simulink model "siso_4_channel_teleop_discrete_wave_PosPos_noise"  (R2021a)
settings: Solver=VariableStepAuto  StartTime=0.0  StopTime=30  FixedStep=Ts  RelTol=1e-3
values from neighbouring files (symbols this model uses):
  A_kalman = [1 Ts ; 0 1 ]    [assignment6.m]
  Amplitude = 1    [assignment6.m]
  b = 1    [assignment6.m]    (also in lessonParams.m)
  Be = 10    [assignment6.m]    (also in lessonParams.m)
  Bh = 1.5    [assignment6.m]    (also in lessonParams.m)
  Bm = 10    [assignment6.m]
  Bs = 30    [assignment6.m]
  C_kalman = [1 0]    [assignment6.m]
  delay = 20    [assignment6.m]
  Dh = 2    [assignment6.m]    (also in lessonParams.m)
  Dm = 0    [assignment6.m]
  Ds = 0    [assignment6.m]
  Fc = 0.1    [assignment6.m]    (also in lessonParams.m = 1)
  Flp = 5    [assignment6.m]
  Ih = 0    [assignment6.m]
  Jh = 0    [assignment6.m]    (also in lessonParams.m = 0.05)
  k_h = 2    [assignment6.m]
  Ke = 200    [assignment6.m]    (also in lessonParams.m)
  Kh = 1    [assignment6.m]    (also in lessonParams.m = 0)
  Km = 50    [assignment6.m]
  Ks = 40    [assignment6.m]
  Mm = 0.5    [assignment6.m]
  Ms = 2    [assignment6.m]
  noiseVariance = 0.00001    (= 1e-05)    [assignment6.m]
  R = 1    [assignment6.m]
  Ts = 0.001    [assignment6.m]    (also in lessonParams.m)
  xe = 0.65    [assignment6.m]
undefined symbols (not defined in the file or in its folder): B, D, DiscIntNeverNeededParam, Discrete, Time
libraries: simulink x4, ctrlSharedLib x2
settings Model: Creator=fabio  LastModifiedBy=fabio

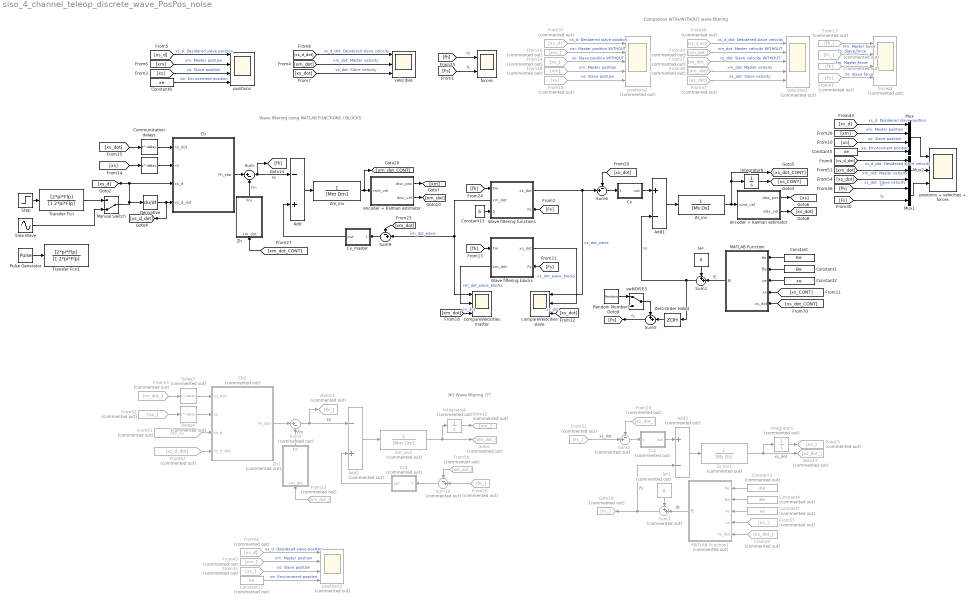
== system siso_4_channel_teleop_discrete_wave_PosPos_noise ==
  note: Wave filtering using MATLAB FUNCTIONS / BLOCKS
  note: Comparison WITH/WITHOUT wave filtering
  note: NO Wave filtering ???
  " " : Delay  DelayLength=delay  SampleTime=Ts
  Add : Sum  Inputs=-+
  Add1 : Sum  Inputs=+-
  Add2 : Sum  Commented=on  Inputs=-+
  Add3 : Sum  Commented=on  Inputs=+-
  Ch : Subsystem
  Ch2 : Subsystem  Commented=on
  Communication delays : Delay  DelayLength=delay  SampleTime=Ts
  Constant : Constant  Value=Ke
  Constant1 : Constant  Value=Be
  Constant11 : Constant  Commented=on  Value=xe
  Constant13 : Constant  Value=b
  Constant2 : Constant  Value=xe
  Constant3 : Constant  Commented=on  Value=Ke
  Constant4 : Constant  Commented=on  Value=Be
  Constant5 : Constant  Value=xe
  Constant6 : Constant  Value=xe
  Constant7 : Constant  Commented=on  Value=xe
  Cv : Subsystem
  Cv1 : Subsystem  Commented=on
  Cv4 : Subsystem  Commented=on
  Cv_master : Subsystem
  Delay3 : Delay  Commented=on  DelayLength=delay  SampleTime=Ts
  Delay4 : Delay  Commented=on  DelayLength=delay  SampleTime=Ts
  Derivative : Derivative
  From17 : From  Commented=on  GotoTag=fh_
  From18 : From  Commented=on  GotoTag=xs
  From{19,29,37,53} (4 alike) : From  Commented=on  GotoTag=xs_dot_
  From22 : From  Commented=on  GotoTag=xm_dot_
  From26 : From  Commented=on  GotoTag=fh_
  From31 : From  Commented=on  GotoTag=Fs_
  From32 : From  Commented=on  GotoTag=Fs_
  From{33..34,52,55} (4 alike) : From  Commented=on  GotoTag=xs_
  From35 : From  Commented=on  GotoTag=xs_d
  From36 : From  Commented=on  GotoTag=xm_
  From38 : From  Commented=on  GotoTag=xm
  From39 : From  Commented=on  GotoTag=xm_dot_
  From40 : From  Commented=on  GotoTag=fh
  From41 : From  Commented=on  GotoTag=Fs
  From42 : From  Commented=on  GotoTag=xs_d
  From45 : From  Commented=on  GotoTag=xm_
  From47 : From  Commented=on  GotoTag=xs_dot
  From48 : From  Commented=on  GotoTag=xs_d_dot
  From49 : From  Commented=on  GotoTag=xm_dot
  From50 : From  Commented=on  GotoTag=xm_dot_
  From61 : From  Commented=on  GotoTag=xs_d
  From62 : From  Commented=on  GotoTag=xs_d_dot
  Goto1 : Goto  Commented=on  GotoTag=xm_dot_
  Goto11 : Goto  Commented=on  GotoTag=fh_
  Goto12 : Goto  Commented=on  GotoTag=xm_
  Goto15 : Goto  Commented=on  GotoTag=xs_
  Goto17 : Goto  Commented=on  GotoTag=xs_dot_
  Goto18 : Goto  Commented=on  GotoTag=Fs_
  Integrator1 : Integrator  Commented=on
  Integrator4 : Integrator  Commented=on
  Integrator6 : Integrator
  MATLAB Function : MATLAB Function  TreatAsAtomicUnit=on
  MATLAB Function1 : MATLAB Function  Commented=on  TreatAsAtomicUnit=on
  Manual Switch : ManualSwitch  CurrentSetting=0
  Mux : Mux
  Mux1 : Mux  Inputs=2
  Mux2 : Mux  Inputs=3
  Pulse Generator : DiscretePulseGenerator  PulseType=Time based  Amplitude=Amplitude  PulseWidth=50  PhaseDelay=1
  Random Number1 : RandomNumber  Variance=noiseVariance  SampleTime=Ts
  Sine Wave : Sin  Amplitude=Amplitude  Frequency=Fc*2*pi  SampleTime=0
  Step : Step  After=Amplitude  SampleTime=0
  Sum : Sum  Inputs=|+-
  Sum1 : Sum  Inputs=++|
  Sum10 : Sum  Commented=on  Inputs=-+|
  Sum2 : Sum  Commented=on  Inputs=|+-
  Sum3 : Sum  Commented=on  Inputs=++|
  Sum4 : Sum  Commented=on  Inputs=-+|
  Sum5 : Sum  Inputs=++|
  Sum6 : Sum  Inputs=-+|
  Sum9 : Sum  Inputs=-+|
  Transfer Fcn : TransferFcn  Numerator=[2*pi*Flp]  Denominator=[1 2*pi*Flp]
  Transfer Fcn1 : TransferFcn  Numerator=[2*pi*Flp]  Denominator=[1 2*pi*Flp]
  Wave filtering blocks : Subsystem
      settings: PortSchema="{\"entries\":[{\"content\":{\"sides\":[{\"content\":{\"connectorIds\":[\"In1\",\"Out2\"]},\"type\":\"ConnectorPlacement.EquallySpacedRectSide\",\"uuid\":\"ee55f81f-a118-497c-9cea-fc8f399218a8\"},{\"content\":{\"connectorIds\":[\"Out1\",\"In2\"],\"side\":\"RIGHT\"},\"type\":\"ConnectorPlacement.EquallySpacedRectSide\",\"uuid\":\"5d1f8501-e1f6-44bf-840d-44d9be1b0103\"},{\"content\":{\"connectorIds\":[],\"side\":\"TOP\"},\"type\":\"ConnectorPlacement.EquallySpacedRectSide\",\"uuid\":\"9e5e7cf5-c9c8-426d-b3a0-7ec1f0160b8f\"}]},\"type\":\"ConnectorPlacement.EquallySpacedConnector\",\"uuid\":\"44941e1b-3958-484a-ae3c-a91d5c4b8d1b\"}],\"packageUris\":[\"http://schema.mathworks.com/mf0/Connector/R2020b\"],\"version\":\"1.0\"}"
  "Wave filtering functions " : Subsystem
      settings: PortSchema="{\"entries\":[{\"content\":{\"sides\":[{\"content\":{\"connectorIds\":[\"In1\",\"Out2\",\"In2\"]},\"type\":\"ConnectorPlacement.EquallySpacedRectSide\",\"uuid\":\"83e83ea2-dad7-4848-b95e-28bc67907647\"},{\"content\":{\"connectorIds\":[\"Out1\",\"In3\"],\"side\":\"RIGHT\"},\"type\":\"ConnectorPlacement.EquallySpacedRectSide\",\"uuid\":\"35e14d6e-ed23-456f-ac9f-64c013712c68\"},{\"content\":{\"connectorIds\":[],\"side\":\"TOP\"},\"type\":\"ConnectorPlacement.EquallySpacedRectSide\",\"uuid\":\"299d1efd-7af2-45ae-8d8e-9fad00b289c8\"}]},\"type\":\"ConnectorPlacement.EquallySpacedConnector\",\"uuid\":\"2f111283-4845-4b8e-bf59-fc37d8c45372\"}],\"packageUris\":[\"http://schema.mathworks.com/mf0/Connector/R2020b\"],\"version\":\"1.0\"}"
  Zero-Order Hold4 : ZeroOrderHold  SampleTime=Ts
  Zh : Subsystem
  Zh1 : Subsystem  Commented=on
  Zm_inv : TransferFcn  Numerator=[0 1]  Denominator=[Mm Dm]
  Zm_inv1 : TransferFcn  Commented=on  Numerator=[0 1]  Denominator=[Mm Dm]
  Zs_inv : TransferFcn  Numerator=[0 1]  Denominator=[Ms Ds]
  Zs_inv1 : TransferFcn  Commented=on  Numerator=[0 1]  Denominator=[Ms Ds]
  "compareVelocities master " : Scope  NumInputPorts=3
  compareVelocities slave : Scope  NumInputPorts=3
  encoder + Kalman estimator : Subsystem
  "encoder + Kalman estimator " : Subsystem
  fe* : Constant  Value=0
  fe*1 : Constant  Commented=on  Value=0
  forces : Scope  NumInputPorts=2
  forces2 : Scope  Commented=on  NumInputPorts=4
  positions : Scope  NumInputPorts=4
  positions + velocities + forces : Scope  NumInputPorts=3
  positions1 : Scope  Commented=on  NumInputPorts=4
  positions2 : Scope  Commented=on  NumInputPorts=5
  swNOISE3 : ManualSwitch
  velocities : Scope  NumInputPorts=3
  velocities1 : Scope  Commented=on  NumInputPorts=5
  wires:
  Zh/1(Fm) -> Sum/2  "Fm"
  Sum/1 -> Add/1, [fh]  "Fh"
  Constant/1 -> MATLAB Function/1(Ke)
  Constant1/1 -> MATLAB Function/2(Be)
  Constant2/1 -> MATLAB Function/3(xe)
  [xs_CONT] -> MATLAB Function/4(xs)
  [xs_dot_CONT] -> MATLAB Function/5(xs_dot)
  MATLAB Function/1(fE) -> Sum1/2  "fE"
  Cv/1(out) -> Add1/1
  Ch/1(Fh_star) -> Sum/1
  [xs_d] -> positions/1  "xs_d: Desidered slave position"
  [xm] -> positions/2  "xm: Master position"
  [xs] -> positions/3  "xs: Slave position"
  [xm_dot] -> velocities/2  "xm_dot: Master velocity"
  [xs_dot] -> velocities/3  "xs_dot: Slave velocity"
  [xs_d_dot] -> velocities/1  "xs_d_dot: Desidered slave velocity"
  Sine Wave/1 -> Manual Switch/2
  Derivative/1 -> [xs_d_dot], Ch/1(xs_d_dot)
  fe*/1 -> Sum1/1
  Step/1 -> Transfer Fcn/1
  Transfer Fcn/1 -> Manual Switch/1
  Manual Switch/1 -> Ch/2(xs_d), [xs_d], Derivative/1
  [xm_dot_CONT] -> Zh/1(xm_dot)
  Constant6/1 -> positions/4  "xe: Environment position"
  [fh] -> forces/1  "fh"
  [Fs] -> forces/2  "fs"
  Pulse Generator/1 -> Transfer Fcn1/1
  [xs_dot] -> Communication delays/1
  Communication delays/1 -> Ch/4(xs_dot)
  [xs] -> " "/1
  " "/1 -> Ch/3(xs)
  [xs_dot] -> Sum6/1
  Sum6/1 -> Cv/1(velErr)
  [xs_dot] -> compareVelocities slave/3  "xs_dot"
  From48/1 -> velocities1/1  "xs_d_dot: Desidered slave velocity"
  From47/1 -> velocities1/5  "xs_dot: Slave velocity"
  From17/1 -> forces2/1  "Fm: Master force"
  From37/1 -> velocities1/3  "xs_dot: Slave velocity WITHOUT"
  From39/1 -> velocities1/2  "xm_dot: Master velocity WITHOUT"
  From40/1 -> forces2/3  "Fm: Master force"
  From18/1 -> positions2/5  "xs: Slave position"
  From35/1 -> positions2/1  "xs_d: Desidered slave position"
  From49/1 -> velocities1/4  "xm_dot: Master velocity"
  From32/1 -> forces2/2  "Fs: Slave force"
  From34/1 -> positions2/3  "xs: Slave position WITHOUT"
  From38/1 -> positions2/4  "xm: Master position"
  From36/1 -> positions2/2  "xm: Master position WITHOUT"
  From41/1 -> forces2/4  "Fs: Slave force"
  Constant11/1 -> positions1/4  "xe: Environment position"
  From33/1 -> positions1/3  "xs: Slave position"
  From45/1 -> positions1/2  "xm: Master position"
  From42/1 -> positions1/1  "xs_d: Desidered slave position"
  Sum1/1 -> Add1/2, Zero-Order Hold4/1  "Fs"
  Sum9/1 -> Cv_master/1(velErr)
  [xm_dot] -> Sum9/1
  [Fs] -> "Wave filtering functions "/3(Fs)
  [fh] -> "Wave filtering functions "/1(Fm)
  Cv_master/1(out) -> Add/2
  Constant13/1 -> "Wave filtering functions "/2(b)
  [fh] -> Wave filtering blocks/1(Fm)
  [Fs] -> Wave filtering blocks/2(Fs)
  Wave filtering blocks/1(xs_dot) -> compareVelocities slave/2  "xs_dot_wave_blocks"
  Wave filtering blocks/2(xm_dot) -> "compareVelocities master "/2  "xm_dot_wave_blocks"
  "Wave filtering functions "/2(xm_dot) -> Sum9/2, "compareVelocities master "/1  "xm_dot_wave"
  "Wave filtering functions "/1(xs_dot) -> Sum6/2, compareVelocities slave/1  "xs_dot_wave"
  From55/1 -> MATLAB Function1/4(xs)
  Integrator1/1 -> Goto15/1
  Cv4/1(out) -> Add2/2
  Ch2/1(Fh_star) -> Sum2/1
  From50/1 -> Sum10/1
  Sum3/1 -> Add3/2, Goto18/1  "Fs"
  From29/1 -> Sum4/1
  Constant7/1 -> MATLAB Function1/3(xe)
  Sum10/1 -> Cv4/1(velErr)
  Sum2/1 -> Add2/1, Goto11/1  "Fh"
  Zm_inv1/1 -> Integrator4/1, Goto1/1
  Cv1/1(out) -> Add3/1
  From19/1 -> MATLAB Function1/5(xs_dot)
  Add3/1 -> Zs_inv1/1
  Add2/1 -> Zm_inv1/1
  Zh1/1(Fm) -> Sum2/2  "Fm"
  Constant3/1 -> MATLAB Function1/1(Ke)
  MATLAB Function1/1(fE) -> Sum3/2  "fE"
  Sum4/1 -> Cv1/1(velErr)
  Constant4/1 -> MATLAB Function1/2(Be)
  Integrator4/1 -> Goto12/1
  From22/1 -> Zh1/1(xm_dot)
  Zs_inv1/1 -> Goto17/1, Integrator1/1  "xs_dot"
  fe*1/1 -> Sum3/1
  Delay3/1 -> Ch2/4(xs_dot)
  From52/1 -> Delay4/1
  From61/1 -> Ch2/2(xs_d)
  From53/1 -> Delay3/1
  Delay4/1 -> Ch2/3(xs)
  From62/1 -> Ch2/1(xs_d_dot)
  From26/1 -> Sum10/2
  From31/1 -> Sum4/2  "xs_dot"
  Add/1 -> Zm_inv/1
  Zm_inv/1 -> [xm_dot_CONT], encoder + Kalman estimator/1(cont_vel)
  encoder + Kalman estimator/1(disc_pos) -> [xm]
  encoder + Kalman estimator/2(disc_vel) -> [xm_dot]
  "encoder + Kalman estimator "/2(disc_vel) -> [xs_dot]
  Integrator6/1 -> [xs_CONT]
  Zs_inv/1 -> Integrator6/1, [xs_dot_CONT], "encoder + Kalman estimator "/1(cont_vel)
  Add1/1 -> Zs_inv/1
  "encoder + Kalman estimator "/1(disc_pos) -> [xs]
  swNOISE3/1 -> Sum5/1
  Random Number1/1 -> swNOISE3/1
  Zero-Order Hold4/1 -> Sum5/2
  Sum5/1 -> [Fs]  "fs"
  [xm_dot] -> "compareVelocities master "/3  "xm_dot"
  Mux1/1 -> positions + velocities + forces/3
  [xs_d_dot] -> Mux2/1  "xs_d_dot: Desidered slave velocity"
  Constant5/1 -> Mux/4  "xe: Environment position"
  Mux/1 -> positions + velocities + forces/1
  Mux2/1 -> positions + velocities + forces/2
  [fh] -> Mux1/1  "fh"
  [xm_dot] -> Mux2/2  "xm_dot: Master velocity"
  [xs] -> Mux/3  "xs: Slave position"
  [xs_dot] -> Mux2/3  "xs_dot: Slave velocity"
  [xm] -> Mux/2  "xm: Master position"
  [xs_d] -> Mux/1  "xs_d: Desidered slave position"
  [Fs] -> Mux1/2  "fs"

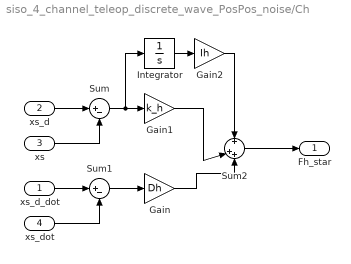
== system siso_4_channel_teleop_discrete_wave_PosPos_noise/Ch ==
  xs_d_dot : Inport
  xs_d : Inport  Port=2
  xs : Inport  Port=3
  xs_dot : Inport  Port=4
  Gain : Gain  Gain=Dh
  Gain1 : Gain  Gain=k_h
  Gain2 : Gain  Gain=Ih
  Integrator : Integrator
  Sum : Sum  Inputs=|+-
  Sum1 : Sum  Inputs=|+-
  Sum2 : Sum  Inputs=+|++
  Fh_star : Outport
  wires:
  Gain1/1 -> Sum2/2
  Sum2/1 -> Fh_star/1
  xs_d/1 -> Sum/1
  xs/1 -> Sum/2
  Sum/1 -> Integrator/1, Gain1/1
  xs_dot/1 -> Sum1/2
  Sum1/1 -> Gain/1
  Gain/1 -> Sum2/3
  xs_d_dot/1 -> Sum1/1
  Integrator/1 -> Gain2/1
  Gain2/1 -> Sum2/1

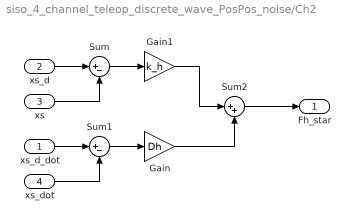
== system siso_4_channel_teleop_discrete_wave_PosPos_noise/Ch2 ==
  xs_d_dot : Inport
  xs_d : Inport  Port=2
  xs : Inport  Port=3
  xs_dot : Inport  Port=4
  Gain : Gain  Gain=Dh
  Gain1 : Gain  Gain=k_h
  Sum : Sum  Inputs=|+-
  Sum1 : Sum  Inputs=|+-
  Sum2 : Sum  Inputs=|++
  Fh_star : Outport
  wires:
  Gain1/1 -> Sum2/1
  Sum2/1 -> Fh_star/1
  xs_d/1 -> Sum/1
  xs/1 -> Sum/2
  Sum/1 -> Gain1/1
  xs_dot/1 -> Sum1/2
  Sum1/1 -> Gain/1
  Gain/1 -> Sum2/2
  xs_d_dot/1 -> Sum1/1

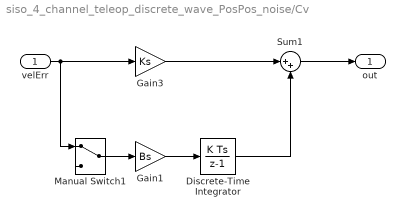
== system siso_4_channel_teleop_discrete_wave_PosPos_noise/Cv ==
  velErr : Inport
  Discrete-Time Integrator : DiscreteIntegrator  SampleTime=-1  ICPrevOutput=DiscIntNeverNeededParam  ICPrevScaledInput=DiscIntNeverNeededParam
  Gain1 : Gain  Gain=Bs
  Gain3 : Gain  Gain=Ks
  Manual Switch1 : ManualSwitch
  Sum1 : Sum  Inputs=|++
  out : Outport
  wires:
  Sum1/1 -> out/1
  Gain3/1 -> Sum1/1
  Gain1/1 -> Discrete-Time Integrator/1
  Discrete-Time Integrator/1 -> Sum1/2
  Manual Switch1/1 -> Gain1/1
  velErr/1 -> Gain3/1, Manual Switch1/1

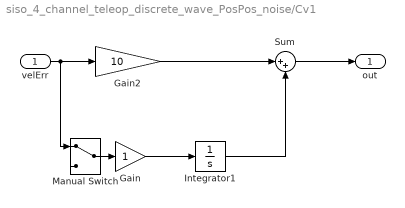
== system siso_4_channel_teleop_discrete_wave_PosPos_noise/Cv1 ==
  velErr : Inport
  Gain : Gain
  Gain2 : Gain  Gain=10
  Integrator1 : Integrator
  Manual Switch : ManualSwitch
  Sum : Sum  Inputs=|++
  out : Outport
  wires:
  velErr/1 -> Manual Switch/1, Gain2/1
  Gain2/1 -> Sum/1
  Sum/1 -> out/1
  Manual Switch/1 -> Gain/1
  Gain/1 -> Integrator1/1
  Integrator1/1 -> Sum/2

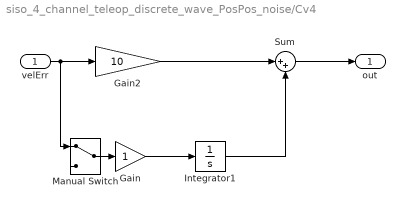
== system siso_4_channel_teleop_discrete_wave_PosPos_noise/Cv4 ==
  velErr : Inport
  Gain : Gain
  Gain2 : Gain  Gain=10
  Integrator1 : Integrator
  Manual Switch : ManualSwitch
  Sum : Sum  Inputs=|++
  out : Outport
  wires:
  velErr/1 -> Manual Switch/1, Gain2/1
  Gain2/1 -> Sum/1
  Sum/1 -> out/1
  Manual Switch/1 -> Gain/1
  Gain/1 -> Integrator1/1
  Integrator1/1 -> Sum/2

== system siso_4_channel_teleop_discrete_wave_PosPos_noise/Cv_master ==
  velErr : Inport
  Discrete-Time Integrator : DiscreteIntegrator  SampleTime=-1  ICPrevOutput=DiscIntNeverNeededParam  ICPrevScaledInput=DiscIntNeverNeededParam
  Gain1 : Gain  Gain=Bm
  Gain3 : Gain  Gain=Km
  Manual Switch1 : ManualSwitch
  Sum1 : Sum  Inputs=|++
  out : Outport
  wires:
  Sum1/1 -> out/1
  Gain3/1 -> Sum1/1
  Gain1/1 -> Discrete-Time Integrator/1
  Manual Switch1/1 -> Gain1/1
  velErr/1 -> Manual Switch1/1, Gain3/1
  Discrete-Time Integrator/1 -> Sum1/2

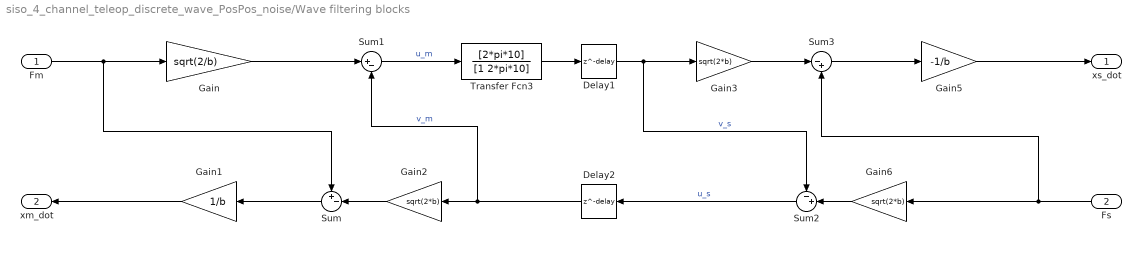
== system siso_4_channel_teleop_discrete_wave_PosPos_noise/Wave filtering blocks ==
  Fm : Inport
  Fs : Inport  Port=2
  Delay1 : Delay  DelayLength=delay  SampleTime=Ts
  Delay2 : Delay  DelayLength=delay  SampleTime=Ts
  Gain : Gain  Gain=sqrt(2/b)
  Gain1 : Gain  Gain=1/b
  Gain2 : Gain  Gain=sqrt(2*b)
  Gain3 : Gain  Gain=sqrt(2*b)
  Gain5 : Gain  Gain=-1/b
  Gain6 : Gain  Gain=sqrt(2*b)
  Sum : Sum  Inputs=+-|
  Sum1 : Sum  Inputs=|+-
  Sum2 : Sum  Inputs=-+|
  Sum3 : Sum  Inputs=|-+
  Transfer Fcn3 : TransferFcn  Numerator=[2*pi*10]  Denominator=[1 2*pi*10]
  xs_dot : Outport
  xm_dot : Outport  Port=2
  wires:
  Sum2/1 -> Delay2/1  "u_s"
  Sum3/1 -> Gain5/1
  Gain/1 -> Sum1/1
  Delay2/1 -> Sum1/2, Gain2/1  "v_m"
  Sum1/1 -> Transfer Fcn3/1  "u_m"
  Gain2/1 -> Sum/2
  Fm/1 -> Sum/1, Gain/1
  Sum/1 -> Gain1/1
  Gain5/1 -> xs_dot/1
  Gain1/1 -> xm_dot/1
  Gain3/1 -> Sum3/1
  Delay1/1 -> Sum2/1, Gain3/1  "v_s"
  Fs/1 -> Gain6/1, Sum3/2
  Gain6/1 -> Sum2/2
  Transfer Fcn3/1 -> Delay1/1

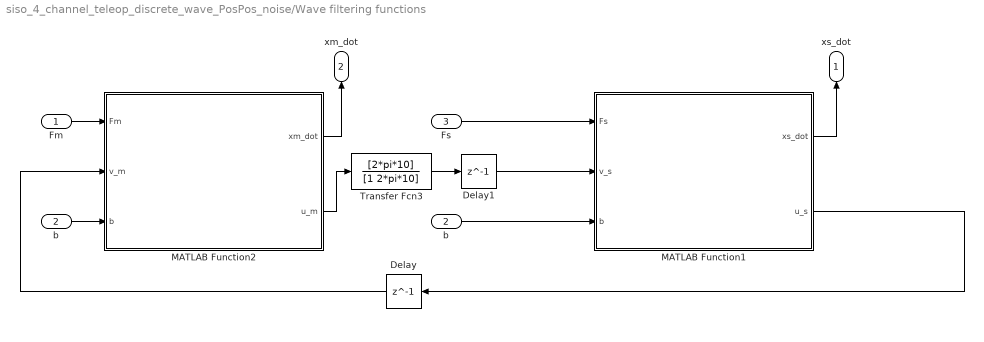
== system siso_4_channel_teleop_discrete_wave_PosPos_noise/Wave filtering functions  ==
  Fm : Inport
  b : Inport  Port=2
  Fs : Inport  Port=3
  Delay : Delay  DelayLength=1  SampleTime=Ts
  Delay1 : Delay  DelayLength=1  SampleTime=Ts
  MATLAB Function1 : MATLAB Function  TreatAsAtomicUnit=on
  MATLAB Function2 : MATLAB Function  TreatAsAtomicUnit=on
  Transfer Fcn3 : TransferFcn  Numerator=[2*pi*10]  Denominator=[1 2*pi*10]
  "b " : InportShadow  Port=2
  xs_dot : Outport
  xm_dot : Outport  Port=2
  wires:
  Delay/1 -> MATLAB Function2/2(v_m)
  b/1 -> MATLAB Function2/3(b)
  Fm/1 -> MATLAB Function2/1(Fm)
  MATLAB Function1/2(u_s) -> Delay/1
  "b "/1 -> MATLAB Function1/3(b)
  Delay1/1 -> MATLAB Function1/2(v_s)
  MATLAB Function1/1(xs_dot) -> xs_dot/1
  MATLAB Function2/1(xm_dot) -> xm_dot/1
  Fs/1 -> MATLAB Function1/1(Fs)
  Transfer Fcn3/1 -> Delay1/1
  MATLAB Function2/2(u_m) -> Transfer Fcn3/1

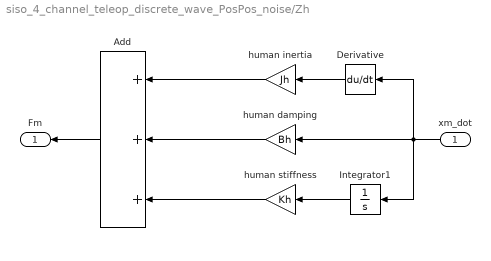
== system siso_4_channel_teleop_discrete_wave_PosPos_noise/Zh ==
  xm_dot : Inport
  Add : Sum  Inputs=+++
  Derivative : Derivative
  Integrator1 : Integrator
  human damping : Gain  Gain=Bh
  human inertia : Gain  Gain=Jh
  human stiffness : Gain  Gain=Kh
  Fm : Outport
  wires:
  Add/1 -> Fm/1
  human stiffness/1 -> Add/3
  human damping/1 -> Add/2
  Integrator1/1 -> human stiffness/1
  xm_dot/1 -> Derivative/1, Integrator1/1, human damping/1
  human inertia/1 -> Add/1
  Derivative/1 -> human inertia/1

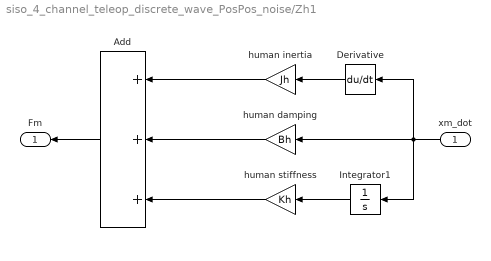
== system siso_4_channel_teleop_discrete_wave_PosPos_noise/Zh1 ==
  xm_dot : Inport
  Add : Sum  Inputs=+++
  Derivative : Derivative
  Integrator1 : Integrator
  human damping : Gain  Gain=Bh
  human inertia : Gain  Gain=Jh
  human stiffness : Gain  Gain=Kh
  Fm : Outport
  wires:
  Add/1 -> Fm/1
  human stiffness/1 -> Add/3
  human damping/1 -> Add/2
  Integrator1/1 -> human stiffness/1
  xm_dot/1 -> Derivative/1, Integrator1/1, human damping/1
  human inertia/1 -> Add/1
  Derivative/1 -> human inertia/1

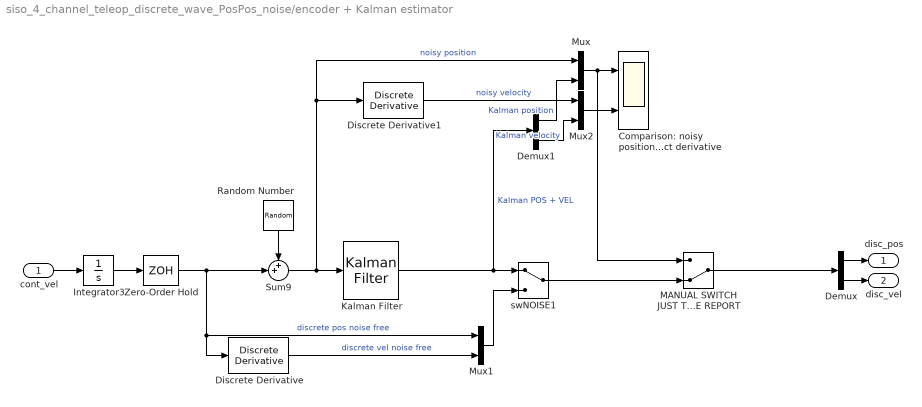
== system siso_4_channel_teleop_discrete_wave_PosPos_noise/encoder + Kalman estimator ==
  cont_vel : Inport
  Comparison: noisy position + Kalman/Direct derivative : Scope  NumInputPorts=2
  Demux : Demux  Outputs=2
  Demux1 : Demux  Outputs=2
  Discrete Derivative : simulink/Discrete/Discrete Derivative  gainval=1.0  ICPrevScaledInput=0.0  OutMin=[]  OutMax=[]  OutDataType=fixdt(1, 16)  OutScaling=2^-10  DoSatur=off
  Discrete Derivative1 : simulink/Discrete/Discrete Derivative  gainval=1.0  ICPrevScaledInput=0.0  OutMin=[]  OutMax=[]  OutDataType=fixdt(1, 16)  OutScaling=2^-10  DoSatur=off
  Integrator3 : Integrator
  Kalman Filter : ctrlSharedLib/Kalman Filter  TimeDomain=Discrete-Time  UseCurrentEstimator=on  ModelSource=Individual A, B, C, D matrices  ModelSourceVariable=sys  A=A_kalman  B=B  C=C_kalman  D=D  NumberOfStates=2  NumberOfInputs=2  NumberOfOutputs=2  InitialEstimateSource=Dialog  X0=0  P0=10  UseK=off  UseGH=off  NumberOfProcessNoiseInputs=2  G=1  TimeInvariantG=on  H=0  TimeInvariantH=on  Q=Q_master  TimeInvariantQ=on  R=R  TimeInvariantR=on  N=0  TimeInvariantN=on  AddInputPort=off  AddEnablePort=off  OutputEstimatedY=off  OutputP=off  Ts=Ts
  MANUAL SWITCH JUST TO PUT INSIDE REPORT : ManualSwitch  CurrentSetting=0
  Mux : Mux  Inputs=2
  Mux1 : Mux  Inputs=2
  Mux2 : Mux  Inputs=2
  Random Number : RandomNumber  Variance=noiseVariance  SampleTime=Ts
  Sum9 : Sum  Inputs=++|
  Zero-Order Hold : ZeroOrderHold  SampleTime=Ts
  swNOISE1 : ManualSwitch
  disc_pos : Outport
  disc_vel : Outport  Port=2
  wires:
  Integrator3/1 -> Zero-Order Hold/1
  cont_vel/1 -> Integrator3/1
  Random Number/1 -> Sum9/1
  Zero-Order Hold/1 -> Discrete Derivative/1, Mux1/1, Sum9/2  "discrete pos noise free"
  Demux/1 -> disc_pos/1
  Demux/2 -> disc_vel/1
  Discrete Derivative/1 -> Mux1/2  "discrete vel noise free"
  Mux1/1 -> swNOISE1/2
  Mux/1 -> MANUAL SWITCH JUST TO PUT INSIDE REPORT/1, Comparison: noisy position + Kalman/Direct derivative/1
  Demux1/2 -> Mux2/2  "Kalman velocity"
  Discrete Derivative1/1 -> Mux2/1  "noisy velocity"
  Kalman Filter/1 -> Demux1/1, swNOISE1/1  "Kalman POS + VEL"
  Sum9/1 -> Mux/1, Discrete Derivative1/1, Kalman Filter/1  "noisy position"
  Demux1/1 -> Mux/2  "Kalman position"
  Mux2/1 -> Comparison: noisy position + Kalman/Direct derivative/2
  MANUAL SWITCH JUST TO PUT INSIDE REPORT/1 -> Demux/1
  swNOISE1/1 -> MANUAL SWITCH JUST TO PUT INSIDE REPORT/2

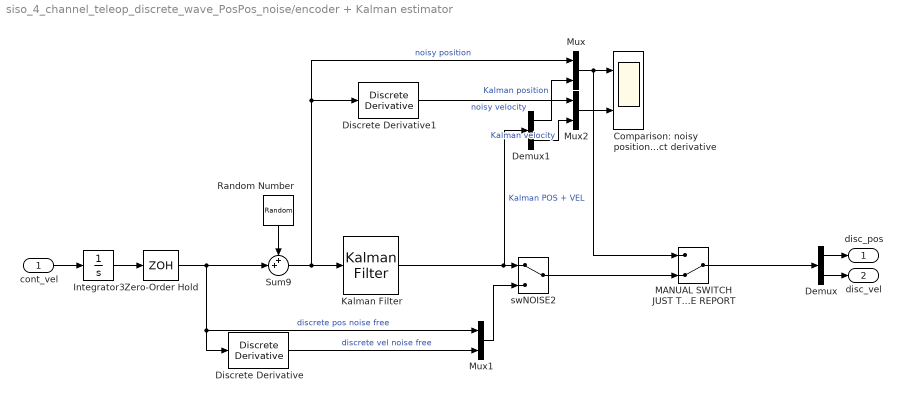
== system siso_4_channel_teleop_discrete_wave_PosPos_noise/encoder + Kalman estimator  ==
  cont_vel : Inport
  Comparison: noisy position + Kalman/Direct derivative : Scope  NumInputPorts=2
  Demux : Demux  Outputs=2
  Demux1 : Demux  Outputs=2
  Discrete Derivative : simulink/Discrete/Discrete Derivative  gainval=1.0  ICPrevScaledInput=0.0  OutMin=[]  OutMax=[]  OutDataType=fixdt(1, 16)  OutScaling=2^-10  DoSatur=off
  Discrete Derivative1 : simulink/Discrete/Discrete Derivative  gainval=1.0  ICPrevScaledInput=0.0  OutMin=[]  OutMax=[]  OutDataType=fixdt(1, 16)  OutScaling=2^-10  DoSatur=off
  Integrator3 : Integrator
  Kalman Filter : ctrlSharedLib/Kalman Filter  TimeDomain=Discrete-Time  UseCurrentEstimator=on  ModelSource=Individual A, B, C, D matrices  ModelSourceVariable=sys  A=A_kalman  B=B  C=C_kalman  D=D  NumberOfStates=2  NumberOfInputs=2  NumberOfOutputs=2  InitialEstimateSource=Dialog  X0=0  P0=10  UseK=off  UseGH=off  NumberOfProcessNoiseInputs=2  G=1  TimeInvariantG=on  H=0  TimeInvariantH=on  Q=Q_master  TimeInvariantQ=on  R=R  TimeInvariantR=on  N=0  TimeInvariantN=on  AddInputPort=off  AddEnablePort=off  OutputEstimatedY=off  OutputP=off  Ts=Ts
  MANUAL SWITCH JUST TO PUT INSIDE REPORT : ManualSwitch  CurrentSetting=0
  Mux : Mux  Inputs=2
  Mux1 : Mux  Inputs=2
  Mux2 : Mux  Inputs=2
  Random Number : RandomNumber  Variance=noiseVariance  SampleTime=Ts
  Sum9 : Sum  Inputs=++|
  Zero-Order Hold : ZeroOrderHold  SampleTime=Ts
  swNOISE2 : ManualSwitch
  disc_pos : Outport
  disc_vel : Outport  Port=2
  wires:
  Integrator3/1 -> Zero-Order Hold/1
  cont_vel/1 -> Integrator3/1
  Random Number/1 -> Sum9/1
  Zero-Order Hold/1 -> Discrete Derivative/1, Mux1/1, Sum9/2  "discrete pos noise free"
  Sum9/1 -> Mux/1, Discrete Derivative1/1, Kalman Filter/1  "noisy position"
  Kalman Filter/1 -> swNOISE2/1, Demux1/1  "Kalman POS + VEL"
  Demux/1 -> disc_pos/1
  Demux/2 -> disc_vel/1
  Discrete Derivative/1 -> Mux1/2  "discrete vel noise free"
  Mux1/1 -> swNOISE2/2
  Mux/1 -> MANUAL SWITCH JUST TO PUT INSIDE REPORT/1, Comparison: noisy position + Kalman/Direct derivative/1
  Demux1/1 -> Mux/2  "Kalman position"
  Mux2/1 -> Comparison: noisy position + Kalman/Direct derivative/2
  Discrete Derivative1/1 -> Mux2/1  "noisy velocity"
  Demux1/2 -> Mux2/2  "Kalman velocity"
  MANUAL SWITCH JUST TO PUT INSIDE REPORT/1 -> Demux/1
  swNOISE2/1 -> MANUAL SWITCH JUST TO PUT INSIDE REPORT/2

== matlab function siso_4_channel_teleop_discrete_wave_PosPos_noise/MATLAB Function1 ==
  data: Ke input; fE output; Be input; xe input; xs input; xs_dot input
function fE = environment(Ke, Be, xe, xs, xs_dot)
    if xs > xe
        fE = Ke*(xs - xe) + Be*xs_dot;
    else
        fE = 0;
    end
end

== matlab function siso_4_channel_teleop_discrete_wave_PosPos_noise/MATLAB Function ==
  data: Ke input; fE output; Be input; xe input; xs input; xs_dot input
function fE = environment(Ke, Be, xe, xs, xs_dot)
    if xs > xe
        fE = Ke*(xs - xe) + Be*xs_dot;
    else
        fE = 0;
    end
end

== matlab function siso_4_channel_teleop_discrete_wave_PosPos_noise/Wave filtering functions /MATLAB Function1 ==
  data: Fs input; xs_dot output; v_s input; u_s output; b input
function [xs_dot, u_s] = wave_fromTo_power_R(Fs, v_s, b)

    u_s = sqrt(2/b)*Fs - v_s;
    xs_dot = -1/b*(Fs - sqrt(2*b)*v_s);
end

== matlab function siso_4_channel_teleop_discrete_wave_PosPos_noise/Wave filtering functions /MATLAB Function2 ==
  data: Fm input; xm_dot output; v_m input; u_m output; b input
function [xm_dot,u_m] = wave_fromTo_power_L(Fm, v_m, b)
    
    u_m = sqrt(2/b)*Fm - v_m;
    xm_dot = 1/b*(Fm - sqrt(2*b)*v_m);

end
